simulink model "Assignment_1_Simulink"  (R2020a)
settings: Solver=FixedStepAuto  StartTime=0.0  StopTime=10.0  FixedStep=1e-3  RelTol=1e-3  EnableMultiTasking=on
undefined symbols (not defined in the file): D0, D1, D10, D11, D12, D13, D2, D3, D4, D5, D6, D7, D8, D9, PTA0, PTA1, PTA2, PTB23, PTB9, PTC16, PTC17, PTC2, PTC3, PTC4, PTD0, PTD1, PTD2, PTD3
libraries: frdmk64flib x15
settings Model: ExtModeTrigDuration=5  Creator=logan_duui82v  LastModifiedBy=logan_duui82v
settings OptimizationCC: EnhancedBackFolding=on  PassReuseOutputArgsAs=Individual arguments  ZeroExternalMemoryAtStartup=off  ZeroInternalMemoryAtStartup=off  MaxStackSize=64  OptimizeBlockOrder=speed  DifferentSizesBufferReuse=on  OptimizationCustomize=off  EfficientTunableParamExpr=on
settings DebuggingCC: ParameterTunabilityLossMsg=error
settings HardwareCC: ProdBitPerPointer=32  ProdBitPerSizeT=32  ProdBitPerPtrDiffT=32  ProdLargestAtomicInteger=Long  ProdLargestAtomicFloat=Double  ProdWordSize=32  ProdHWDeviceType=ARM Compatible->ARM Cortex
settings SFSimCC: MATLABDynamicMemAlloc=off
settings RTWCC: SystemTargetFile=ert.tlc  HardwareBoard=NXP FRDM-K64F  TemplateMakefile=ert_default_tmf  Toolchain=GNU Tools for ARM Embedded Processors
settings CodeAppCC: ForceParamTrailComments=on  IgnoreCustomStorageClasses=off  OperatorAnnotations=on  SimulinkDataObjDesc=on  SFDataObjDesc=on  InsertBlockDesc=on

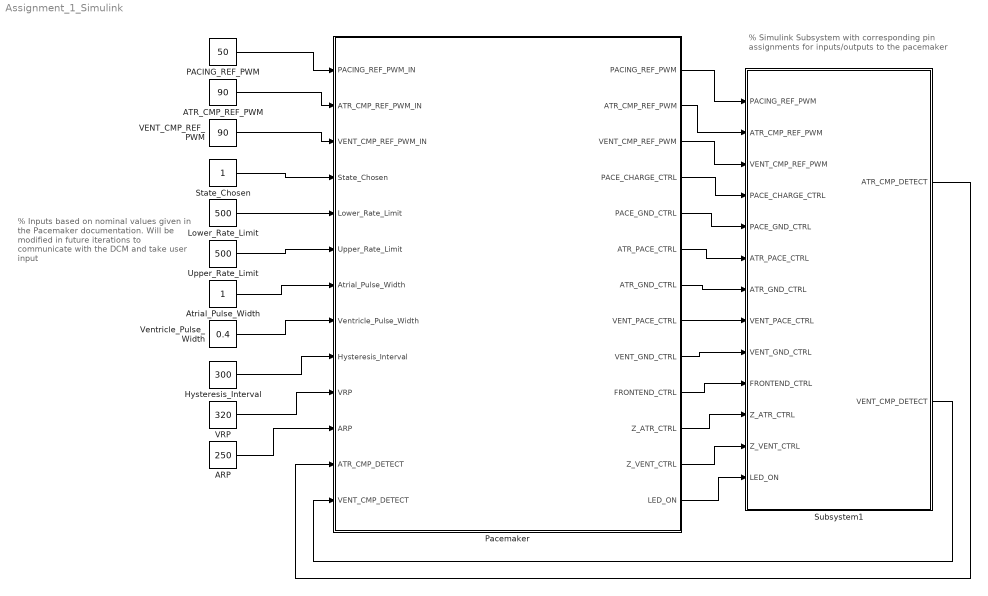
== system Assignment_1_Simulink ==
  note: % Inputs based on nominal values
      | given in the Pacemaker documentation.
      | Will be modified in future iterations to
      | communicate with the DCM and take
      | user input
  note: % Simulink Subsystem with corresponding pin
      | assignments for inputs/outputs to the pacemaker
  ARP : Constant  Value=250
  ATR_CMP_REF_PWM : Constant  Value=90
  Atrial_Pulse_Width : Constant  OutDataTypeStr=int32
  Hysteresis_Interval : Constant  Value=300  OutDataTypeStr=int32
  Lower_Rate_Limit : Constant  Value=500  OutDataTypeStr=int32
  PACING_REF_PWM : Constant  Value=50  OutDataTypeStr=double
  Pacemaker : Stateflow chart  TreatAsAtomicUnit=on
      settings: PortSchema="{\"entries\":[{\"content\":{\"sides\":[{\"content\":{\"connectorIds\":[\"In11\",\"In12\",\"In13\",\"In3\",\"In1\",\"In4\",\"In2\",\"In6\",\"In8\",\"In9\",\"In10\",\"In5\",\"In7\"]},\"type\":\"ConnectorPlacement.EquallySpacedRectSide\",\"uuid\":\"df877ca0-8245-4163-8fee-7182eab1d55d\"},{\"content\":{\"connectorIds\":[\"Out11\",\"Out12\",\"Out13\",\"Out2\",\"Out3\",\"Out1\",\"Out5\",\"Out7\",\"Out8\",\"Out10\",\"Out4\",\"Out9\",\"Out6\"],\"side\":\"RIGHT\"},\"type\":\"ConnectorPlacement.EquallySpacedRectSide\",\"uuid\":\"3a694184-6a85-4729-834f-a3ab7480664d\"},{\"content\":{\"connectorIds\":[],\"side\":\"TOP\"},\"type\":\"ConnectorPlacement.EquallySpacedRectSide\",\"uuid\":\"45b3d390-d3d3-4e22-8b52-b1590054c23a\"}]},\"type\":\"ConnectorPlacement.EquallySpacedConnector\",\"uuid\":\"ad3b7ed4-c882-4247-8e15-d6beb1b6e9a6\"}],\"packageUris\":[\"http://schema.mathworks.com/mf0/Connector/19700101\"],\"version\":\"1.0\"}"
  State_Chosen : Constant  OutDataTypeStr=int32
  Subsystem1 : Subsystem
  Upper_Rate_Limit : Constant  Value=500  OutDataTypeStr=int32
  VENT_CMP_REF_PWM : Constant  Value=90
  VRP : Constant  Value=320
  Ventricle_Pulse_Width : Constant  Value=0.4  OutDataTypeStr=int32
  wires:
  State_Chosen/1 -> Pacemaker/3(State_Chosen)
  Atrial_Pulse_Width/1 -> Pacemaker/2(Atrial_Pulse_Width)
  Lower_Rate_Limit/1 -> Pacemaker/1(Lower_Rate_Limit)
  Upper_Rate_Limit/1 -> Pacemaker/4(Upper_Rate_Limit)
  Pacemaker/6(LED_ON) -> Subsystem1/13(LED_ON)
  Subsystem1/1(ATR_CMP_DETECT) -> Pacemaker/5(ATR_CMP_DETECT)
  Subsystem1/2(" VENT_CMP_DETECT") -> Pacemaker/7(VENT_CMP_DETECT)
  Hysteresis_Interval/1 -> Pacemaker/8(Hysteresis_Interval)
  Ventricle_Pulse_Width/1 -> Pacemaker/6(Ventricle_Pulse_Width)
  Pacemaker/9(Z_VENT_CTRL) -> Subsystem1/12(Z_VENT_CTRL)
  Pacemaker/4(Z_ATR_CTRL) -> Subsystem1/11(Z_ATR_CTRL)
  Pacemaker/10(FRONTEND_CTRL) -> Subsystem1/10(FRONTEND_CTRL)
  Pacemaker/8(VENT_GND_CTRL) -> Subsystem1/9(VENT_GND_CTRL)
  Pacemaker/7(VENT_PACE_CTRL) -> Subsystem1/8(VENT_PACE_CTRL)
  Pacemaker/2(PACE_CHARGE_CTRL) -> Subsystem1/4(PACE_CHARGE_CTRL)
  Pacemaker/3(PACE_GND_CTRL) -> Subsystem1/5(PACE_GND_CTRL)
  Pacemaker/1(ATR_PACE_CTRL) -> Subsystem1/6(ATR_PACE_CTRL)
  Pacemaker/5(ATR_GND_CTRL) -> Subsystem1/7(ATR_GND_CTRL)
  PACING_REF_PWM/1 -> Pacemaker/11(PACING_REF_PWM_IN)
  ATR_CMP_REF_PWM/1 -> Pacemaker/12(ATR_CMP_REF_PWM_IN)
  VENT_CMP_REF_PWM/1 -> Pacemaker/13(VENT_CMP_REF_PWM_IN)
  VRP/1 -> Pacemaker/9(VRP)
  ARP/1 -> Pacemaker/10(ARP)
  Pacemaker/11(PACING_REF_PWM) -> Subsystem1/1(PACING_REF_PWM)
  Pacemaker/12(ATR_CMP_REF_PWM) -> Subsystem1/2(ATR_CMP_REF_PWM)
  Pacemaker/13(VENT_CMP_REF_PWM) -> Subsystem1/3(VENT_CMP_REF_PWM)

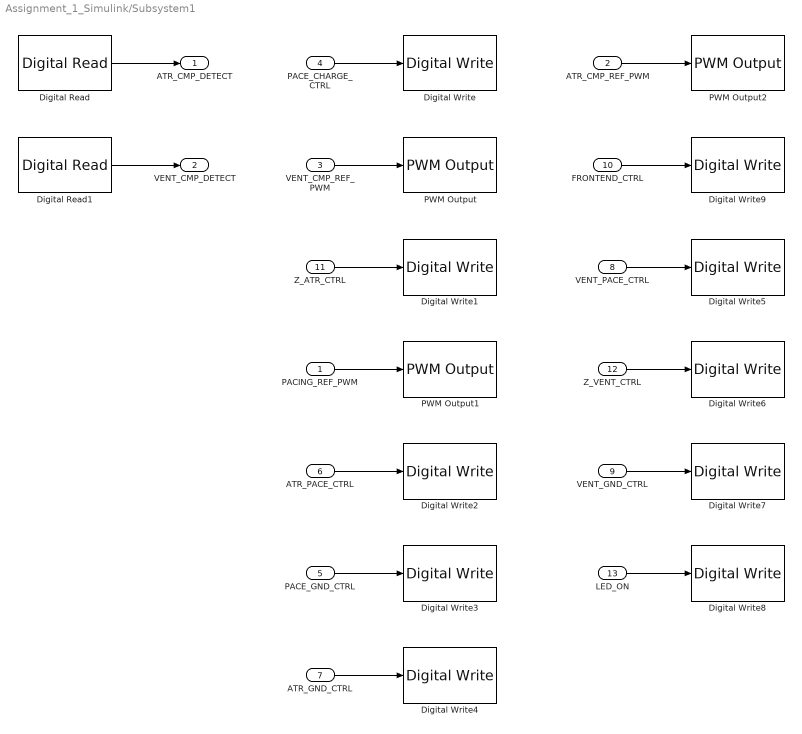
== system Assignment_1_Simulink/Subsystem1 ==
  PACING_REF_PWM : Inport
  ATR_CMP_REF_PWM : Inport  Port=2
  VENT_CMP_REF_PWM : Inport  Port=3
  PACE_CHARGE_CTRL : Inport  Port=4
  PACE_GND_CTRL : Inport  Port=5
  ATR_PACE_CTRL : Inport  Port=6
  ATR_GND_CTRL : Inport  Port=7
  VENT_PACE_CTRL : Inport  Port=8
  VENT_GND_CTRL : Inport  Port=9
  FRONTEND_CTRL : Inport  Port=10
  Z_ATR_CTRL : Inport  Port=11
  Z_VENT_CTRL : Inport  Port=12
  LED_ON : Inport  Port=13
  Digital Read : frdmk64flib/Digital Read  Whichpin=PTC16 (D0)  SampleTime=-1
  Digital Read1 : frdmk64flib/Digital Read  Whichpin=PTC17 (D1)  SampleTime=-1
  Digital Write : frdmk64flib/Digital Write  Whichpin=PTB9 (D2)
  Digital Write1 : frdmk64flib/Digital Write  Whichpin=PTB23 (D4)
  Digital Write2 : frdmk64flib/Digital Write  Whichpin=PTA0 (D8)
  Digital Write3 : frdmk64flib/Digital Write  Whichpin=PTD0 (D10)
  Digital Write4 : frdmk64flib/Digital Write  Whichpin=PTD2 (D11)
  Digital Write5 : frdmk64flib/Digital Write  Whichpin=PTC4 (D9)
  Digital Write6 : frdmk64flib/Digital Write  Whichpin=PTC3 (D7)
  Digital Write7 : frdmk64flib/Digital Write  Whichpin=PTD3 (D12)
  Digital Write8 : frdmk64flib/Digital Write  Whichpin=RED_LED
  Digital Write9 : frdmk64flib/Digital Write  Whichpin=PTD1 (D13)
  PWM Output : frdmk64flib/PWM Output  Whichpin=PTA1 (D3)  InitialFrequency=2000  InitialDutyCycle=100
  PWM Output1 : frdmk64flib/PWM Output  Whichpin=PTA2 (D5)  InitialFrequency=2000  InitialDutyCycle=50
  PWM Output2 : frdmk64flib/PWM Output  Whichpin=PTC2 (D6)  InitialFrequency=2000  InitialDutyCycle=100
  ATR_CMP_DETECT : Outport
  " VENT_CMP_DETECT" : Outport  Port=2
  wires:
  Digital Read/1 -> ATR_CMP_DETECT/1
  Digital Read1/1 -> " VENT_CMP_DETECT"/1
  PACE_CHARGE_CTRL/1 -> Digital Write/1
  VENT_CMP_REF_PWM/1 -> PWM Output/1
  Z_ATR_CTRL/1 -> Digital Write1/1
  PACING_REF_PWM/1 -> PWM Output1/1
  ATR_PACE_CTRL/1 -> Digital Write2/1
  PACE_GND_CTRL/1 -> Digital Write3/1
  ATR_GND_CTRL/1 -> Digital Write4/1
  VENT_PACE_CTRL/1 -> Digital Write5/1
  Z_VENT_CTRL/1 -> Digital Write6/1
  VENT_GND_CTRL/1 -> Digital Write7/1
  LED_ON/1 -> Digital Write8/1
  ATR_CMP_REF_PWM/1 -> PWM Output2/1
  FRONTEND_CTRL/1 -> Digital Write9/1

== stateflow chart Assignment_1_Simulink/Pacemaker ==
  state AOO
    state ChargingDischarging
      entry:
      %No Sensing
      FRONTEND_CTRL = false;
      %Charging
      PACE_CHARGE_CTRL = true;
      ATR_PACE_CTRL = false;
      VENT_PACE_CTRL = false;
      %Discharging
      PACE_GND_CTRL = true;
      ATR_PACE_CTRL = false;
      ATR_GND_CTRL = true;
      VENT_PACE_CTRL = false;
      VENT_GND_CTRL = false;
      Z_ATR_CTRL = false;
      Z_VENT_CTRL = false;
      LED_ON = false;
    state APacing
      entry:
      %Pace Atrial
      PACE_CHARGE_CTRL = false;
      PACE_GND_CTRL = true;
      ATR_PACE_CTRL = true;
      ATR_GND_CTRL = false;
      VENT_PACE_CTRL = false;
      VENT_GND_CTRL = false;
      Z_ATR_CTRL = false;
      Z_VENT_CTRL = false;
      LED_ON = true;
    note: % Charges until after the lower rate limit
        | passes, sends a pulse for as long as the
        | pulse width. Cycle repeats.
    (default) -> AOO.ChargingDischarging
    AOO.ChargingDischarging -> AOO.APacing : [after(Lower_Rate_Limit - Atrial_Pulse_Width, msec)]
    AOO.APacing -> AOO.ChargingDischarging : [after(Atrial_Pulse_Width,msec)]
  state VOO
    state ChargingDischarging
      entry:
      %No Sensing
      FRONTEND_CTRL = false;
      %Charging
      PACE_CHARGE_CTRL = true;
      ATR_PACE_CTRL = false;
      VENT_PACE_CTRL = false;
      %Discharging
      PACE_GND_CTRL = true;
      ATR_PACE_CTRL = false;
      ATR_GND_CTRL = false;
      VENT_PACE_CTRL = false;
      VENT_GND_CTRL = true;
      Z_ATR_CTRL = false;
      Z_VENT_CTRL = false;
      LED_ON = false;
    state VPacing
      entry:
      %Pace Ventricle
      PACE_CHARGE_CTRL = false;
      PACE_GND_CTRL = true;
      ATR_PACE_CTRL = false;
      ATR_GND_CTRL = false;
      VENT_PACE_CTRL = true;
      VENT_GND_CTRL = false;
      Z_ATR_CTRL = false;
      Z_VENT_CTRL = false;
      LED_ON = true;
    (default) -> VOO.ChargingDischarging
    VOO.ChargingDischarging -> VOO.VPacing : [after(Lower_Rate_Limit, msec)]
    VOO.VPacing -> VOO.ChargingDischarging : [after(Ventricle_Pulse_Width,msec)]
  state AAI
    state APacing
      entry:
      %Disable Sensing
      FRONTEND_CTRL = false;
      %Pace Atrial
      PACE_CHARGE_CTRL = false;
      PACE_GND_CTRL = true;
      ATR_PACE_CTRL = true;
      ATR_GND_CTRL = false;
      VENT_PACE_CTRL = false;
      VENT_GND_CTRL = false;
      Z_ATR_CTRL = false;
      Z_VENT_CTRL = false;
      LED_ON = true;
    state ChargingDischarging
      entry:
      %Enable Sensing
      FRONTEND_CTRL = true;
      %Charging
      PACE_CHARGE_CTRL = true;
      ATR_PACE_CTRL = false;
      VENT_PACE_CTRL = false;
      %Discharging
      PACE_GND_CTRL = true;
      ATR_PACE_CTRL = false;
      ATR_GND_CTRL = true;
      VENT_PACE_CTRL = false;
      VENT_GND_CTRL = false;
      Z_ATR_CTRL = false;
      Z_VENT_CTRL = false;
      LED_ON = false;
    state Hysteresis
      entry:
      %Enable Sensing
      FRONTEND_CTRL = true;
      %Charging
      PACE_CHARGE_CTRL = true;
      ATR_PACE_CTRL = false;
      VENT_PACE_CTRL = false;
      %Discharging
      PACE_GND_CTRL = true;
      ATR_PACE_CTRL = false;
      ATR_GND_CTRL = true;
      VENT_PACE_CTRL = false;
      VENT_GND_CTRL = false;
      Z_ATR_CTRL = false;
      Z_VENT_CTRL = false;
      LED_ON = false;
    note: % If a natural heart beat is detected,
        | enter the Hysteresis state until no
        | natural beat occurs for the lower rate
        | limit plus the hysteresis interval
    (default) -> AAI.ChargingDischarging
    AAI.ChargingDischarging -> AAI.APacing [order 1] : [after(Lower_Rate_Limit - Atrial_Pulse_Width, msec)]
    AAI.APacing -> AAI.ChargingDischarging : [after(Atrial_Pulse_Width,msec)]
    AAI.Hysteresis -> AAI.APacing [order 1] : [after(Lower_Rate_Limit + Hysteresis_Interval, msec)]
    AAI.ChargingDischarging -> AAI.Hysteresis [order 2] : [after(ARP, msec) && ATR_CMP_DETECT == true]
    AAI.Hysteresis -> AAI.Hysteresis [order 2] : [after(ARP, msec) && ATR_CMP_DETECT == true]
  state VVI
    state ChargingDischarging
      entry:
      %Enable Sensing
      FRONTEND_CTRL = true;
      %Charging
      PACE_CHARGE_CTRL = true;
      ATR_PACE_CTRL = false;
      VENT_PACE_CTRL = false;
      %Discharging
      PACE_GND_CTRL = true;
      ATR_PACE_CTRL = false;
      ATR_GND_CTRL = false;
      VENT_PACE_CTRL = false;
      VENT_GND_CTRL = true;
      Z_ATR_CTRL = false;
      Z_VENT_CTRL = false;
      LED_ON = false;
    state VPacing
      entry:
      %Disable Sensing
      FRONTEND_CTRL = false;
      %Pace Ventricle
      PACE_CHARGE_CTRL = false;
      PACE_GND_CTRL = true;
      ATR_PACE_CTRL = false;
      ATR_GND_CTRL = false;
      VENT_PACE_CTRL = true;
      VENT_GND_CTRL = false;
      Z_ATR_CTRL = false;
      Z_VENT_CTRL = false;
      LED_ON = true;
    state Hysteresis
      entry:
      %Enable Sensing
      FRONTEND_CTRL = true;
      %Charging
      PACE_CHARGE_CTRL = true;
      ATR_PACE_CTRL = false;
      VENT_PACE_CTRL = false;
      %Discharging
      PACE_GND_CTRL = true;
      ATR_PACE_CTRL = false;
      ATR_GND_CTRL = false;
      VENT_PACE_CTRL = false;
      VENT_GND_CTRL = true;
      Z_ATR_CTRL = false;
      Z_VENT_CTRL = false;
      LED_ON = false;
    (default) -> VVI.ChargingDischarging
    VVI.ChargingDischarging -> VVI.VPacing [order 1] : [after(Lower_Rate_Limit - Ventricle_Pulse_Width, msec)]
    VVI.VPacing -> VVI.ChargingDischarging : [after(Ventricle_Pulse_Width,msec)]
    VVI.Hysteresis -> VVI.VPacing [order 2] : [after(Lower_Rate_Limit + Hysteresis_Interval, msec)]
    VVI.ChargingDischarging -> VVI.Hysteresis [order 2] : [after(VRP, msec) && VENT_CMP_DETECT==true]
    VVI.Hysteresis -> VVI.Hysteresis [order 1] : [after(VRP, msec) && VENT_CMP_DETECT==true]
  state initialState
  note: % Upon startup, pacemaker goes into the selected
      | mode based on the "State_Chosen" variable
  initialState -> AOO [order 1] : [State_Chosen==1]
  initialState -> VOO [order 2] : [State_Chosen==2]
  initialState -> AAI [order 3] : [State_Chosen==3]
  initialState -> VVI [order 4] : [State_Chosen==4]
  (default) -> initialState
  data: Lower_Rate_Limit input int32; Atrial_Pulse_Width input int32; State_Chosen input int32; Upper_Rate_Limit input; ATR_PACE_CTRL output boolean =false; PACE_CHARGE_CTRL output boolean =false; PACE_GND_CTRL output boolean =false; Z_ATR_CTRL output boolean =false; ATR_GND_CTRL output boolean =false; LED_ON output boolean; VENT_PACE_CTRL output boolean; VENT_GND_CTRL output; Z_VENT_CTRL output; ATR_CMP_DETECT input boolean; Ventricle_Pulse_Width input int32; VENT_CMP_DETECT input; Hysteresis_Interval input int32; FRONTEND_CTRL output; VRP input; ARP input; PACING_REF_PWM output; ATR_CMP_REF_PWM output; VENT_CMP_REF_PWM output; PACING_REF_PWM_IN input; ATR_CMP_REF_PWM_IN input; VENT_CMP_REF_PWM_IN input
